simulink model "demo2_supervisory"  (R2024b)
settings: Solver=FixedStepAuto  StartTime=0.0  StopTime=3/60  FixedStep=1/12000  RelTol=1e-3
undefined symbols (not defined in the file): Fault_Inv, GA_th_2, SW, Vd_max, Vd_min, Vdc1, Vdc2, Vdc3, Vdc4, Vdc5, Vq_max, Vq_min
libraries: spsDCVoltageSourceLib x5, spsFullBridgeConverterLib x5, spsSeriesRLCBranchLib x1, spsAlphaBetaZerotodq0Lib x1, spsMeanLib x1, simulink x1, spsVoltageMeasurementLib x1, spspowerguiLib x1
(part 1 of 2)
settings Model: Creator=pgm
settings DataIOCC: ReturnWorkspaceOutputs=off
settings ModelReferenceCC: EnableRefExpFcnMdlSchedulingChecks=on
settings RTWCC: GPUComputeCapability=3.5

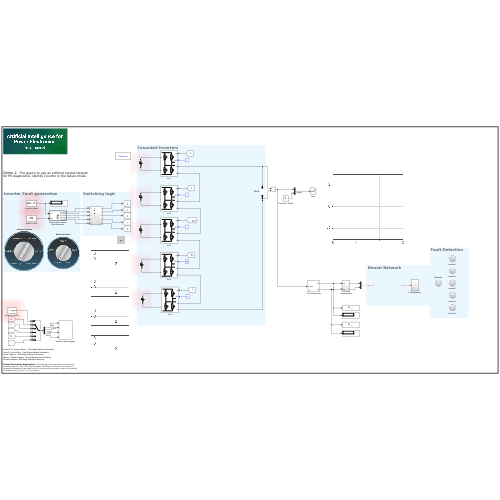
[thumbnail: Simulink's stored preview of the top-level diagram]
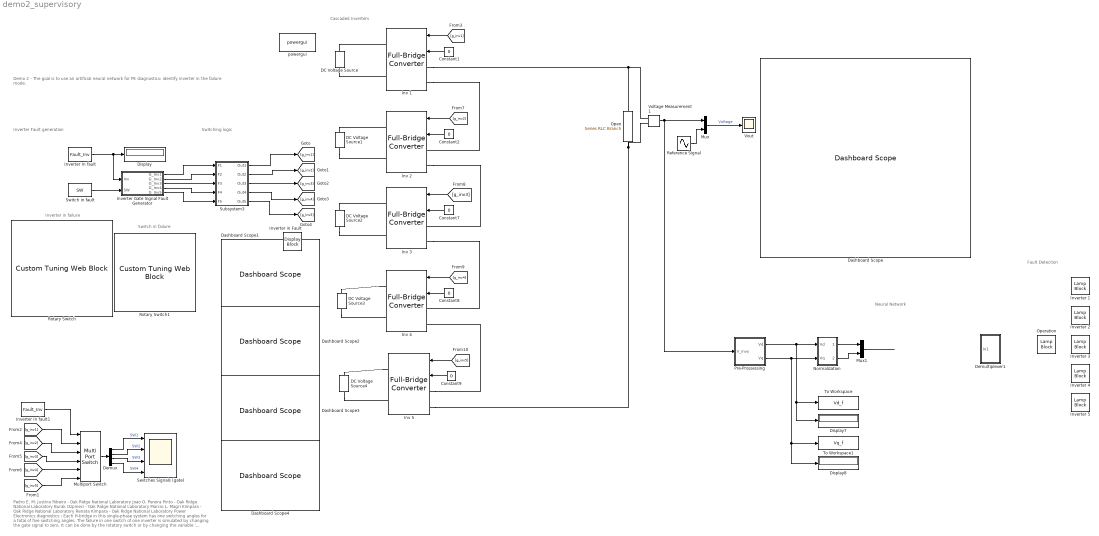
== system demo2_supervisory ==
  note: Inverter in failure
  note: Neural Network
  note: Switching logic
  note: Cascaded Inverters
  note: Inverter Fault generation
  note: Fault Detection
  note: Demo 2 - The goal is to use an artificial neural network for PE diagnostics: identify inverter in the failure mode.
  note: Switch in failure
  note: Pedro E. M. Justino Ribeiro - Oak Ridge National Laboratory
      | Joao O. Pereira Pinto - Oak Ridge National Laboratory
      | Burak Ozpineci - Oak Ridge National Laboratory
      | Marcio L. Magri Kimpara - Oak Ridge National Laboratory
      | Renata Kimpara - Oak Ridge National Laboratory
      |
      | Power Electronics diagnostics : Each H-bridge in this single-phase system has one switching angles for a total of five switching angles. The failure in one switch of one inverter is simulated by changing the gate signal to zero. It can be done by the rotatory switch or by changing the variable ' Fault_Inv' from 1 to 5 in workspace.
  Constant{1..2,7..9} (5 alike) : Constant  Value=0
  DC Voltage Source : spsDCVoltageSourceLib/DC Voltage Source  Amplitude=Vdc1  Measurements=None
  DC Voltage Source1 : spsDCVoltageSourceLib/DC Voltage Source  Amplitude=Vdc2  Measurements=None
  DC Voltage Source2 : spsDCVoltageSourceLib/DC Voltage Source  Amplitude=Vdc3  Measurements=None
  DC Voltage Source3 : spsDCVoltageSourceLib/DC Voltage Source  Amplitude=Vdc4  Measurements=None
  DC Voltage Source4 : spsDCVoltageSourceLib/DC Voltage Source  Amplitude=Vdc5  Measurements=None
  Dashboard Scope : DashboardScope
  Dashboard Scope{1..4} (4 alike) : DashboardScope  TicksPosition=Inside
  Demultiplexer1 : Subsystem
  Demux : Demux
  Display : Display
  Display7 : Display
      settings: Format=short_e
  Display8 : Display
      settings: Format=short_e
  Inv {1..5} (5 alike) : spsFullBridgeConverterLib/Full-Bridge Converter  ModelType=Switching devices  Ron=1e-3  Rs=1e6  Cs=inf  Vforward=[0,0]  Ron_Diode=1e-3  Rs_Diode=1e6  Cs_Diode=inf  Vf_Diode=1e-3  Rs_CurrentSource=inf  Ron_ACsource=1e-3
  Inverter {1..5} (5 alike) : LampBlock  LabelPosition=Hide
  Inverter Gate Signal Fault Generator : MATLAB Function  TreatAsAtomicUnit=on
  Inverter In fault : Constant  Value=Fault_Inv
  Inverter In fault1 : Constant  Value=Fault_Inv
  Inverter in Fault : DisplayBlock  LabelPosition=Hide  Transparency=1
  Multiport Switch : MultiPortSwitch  Inputs=5  DiagnosticForDefault=None  SaturateOnIntegerOverflow=off  InputSameDT=off
  Mux : Mux  Inputs=2
  Mux1 : Mux  Inputs=2
  Normalization : Subsystem
  Open : spsSeriesRLCBranchLib/Series RLC Branch  LConnTagsString=__new0  RConnTagsString=__new0  BranchType=Open circuit  Resistance=50  Inductance=3e-3  SetiL0=off  InitialCurrent=0  Capacitance=400e-6  Setx0=off  InitialVoltage=0  Measurements=None
  "Operation " : LampBlock  LabelPosition=Hide
  Pre-Prossessing : Subsystem  mask{Parameter1=}
      mask prompts: Parameter1 "Transformation"
  Reference Signal : Sin  Amplitude=120*sqrt(2)  Frequency=2*pi*60  SampleTime=0
  Rotary Switch : CustomTuningWebBlock  LabelPosition=Hide  ShowInitialText=on  Configuration="{\"components\":[{\"name\":\"RotarySwitchComponent\",\"settings\":{\"arcAngle\":300,\"arcAngleOffset\":120,\"handle\":{\"size\":[150,150],\"src\":\"data:image\\/svg+xml;base64,PHN2ZyBpZD0iTGF5ZXJfMSIgZGF0YS1uYW1lPSJMYXllciAxIiB4bWxucz0iaHR0cDovL3d3dy53My5vcmcvMjAwMC9zdmciIHhtbG5zOnhsaW5rPSJodHRwOi8vd3d3LnczLm9yZy8xOTk5L3hsaW5rIiB2aWV3Qm94PSIwIDAgMTIxIDEyMSI+PGRlZnM+PHN0eWxlPi5jbHMtMXtmaWxsOnVybCgjbGluZWFyLWdyYWRpZW50KTt9LmNscy0yLC5jbHMtM3tmaWxsOiNkMWQxZDE7fS5jbHMtM3tzdHJva2U6I2I3YjdiNztzdHJva2UtbWl0ZXJsaW1pdDoxMDtzdHJva2Utd2lkdGg6MC4yNXB4O30uY2xzLTR7ZmlsbDojZjMwMDAwO30uY2xzLTV7ZmlsbDojZjIxNzY3O308L3N0eWxlPjxsaW5lYXJHcmFkaWVudCBpZD0ibGluZWFyLWdyYWRpZW50IiB4MT0iNjAuNSIgeTE9IjEyMC41IiB4Mj0iNjAuNSIgeTI9IjAuNSIgZ3JhZGllbnRVbml0cz0idXNlclNwYWNlT25Vc2UiPjxzdG9wIG9mZnNldD0iMCIgc3RvcC1jb2xvcj0iI2QxZDFkMSIvPjxzdG9wIG9mZnNldD0iMC4xIiBzdG9wLWNvbG9yPSIjY2VjZWNlIi8+PHN0b3Agb2Zmc2V0PSIwLjE5IiBzdG9wLWNvbG9yPSIjYzNjM2MzIi8+PHN0b3Agb2Zmc2V0PSIwLjI4IiBzdG9wLWNvbG9yPSIjYjFiMWIxIi8+PHN0b3Agb2Zmc2V0PSIwLjM2IiBzdG9wLWNvbG9yPSIjOTg5ODk4Ii8+PHN0b3Agb2Zmc2V0PSIwLjQ0IiBzdG9wLWNvbG9yPSIjNzg3ODc4Ii8+PHN0b3Agb2Zmc2V0PSIwLjQ2IiBzdG9wLWNvbG9yPSIjNmI2YjZiIi8+PHN0b3Agb2Zmc2V0PSIwLjU0IiBzdG9wLWNvbG9yPSIjNmI2YjZiIi8+PHN0b3Agb2Zmc2V0PSIwLjU2IiBzdG9wLWNvbG9yPSIjNzY3Njc2Ii8+PHN0b3Agb2Zmc2V0PSIwLjY0IiBzdG9wLWNvbG9yPSIjOTc5Nzk3Ii8+PHN0b3Agb2Zmc2V0PSIwLjcyIiBzdG9wLWNvbG9yPSIjYjBiMGIwIi8+PHN0b3Agb2Zmc2V0PSIwLjgxIiBzdG9wLWNvbG9yPSIjYzNjM2MzIi8+PHN0b3Agb2Zmc2V0PSIwLjkiIHN0b3AtY29sb3I9IiNjZGNkY2QiLz48c3RvcCBvZmZzZXQ9IjEiIHN0b3AtY29sb3I9IiNkMWQxZDEiLz48L2xpbmVhckdyYWRpZW50PjwvZGVmcz48Y2lyY2xlIGNsYXNzPSJjbHMtMSIgY3g9IjYwLjUiIGN5PSI2MC41IiByPSI2MCIvPjxwYXRoIGNsYXNzPSJjbHMtMiIgZD0iTTYwLjUsMUE1OS41LDU5LjUsMCwxLDEsMSw2MC41LDU5LjU3LDU5LjU3LDAsMCwxLDYwLjUsMW0wLTFBNjAuNSw2MC41LDAsMSwwLDEyMSw2MC41LDYwLjUsNjAuNSwwLDAsMCw2MC41LDBaIi8+PHJlY3QgY2xhc3M9ImNscy0zIiB4PSIwLjUiIHk9IjUxLjUiIHdpZHRoPSIxMjAiIGhlaWdodD0iMTgiIHJ4PSIzLjA0Ii8+PHJlY3QgY2xhc3M9ImNscy00IiB4PSI1Ljc1IiB5PSI1OC43NSIgd2lkdGg9IjE2IiBoZWlnaHQ9IjMiLz48cGF0aCBjbGFzcz0iY2xzLTUiIGQ9Ik0yMS4yNSw1OS4yNXYyaC0xNXYtMmgxNW0xLTFoLTE3djRoMTd2LTRaIi8+PC9zdmc+\"},\"handleOffset\":[0.00839802927552135,0],\"handleOrientation\":180,\"handlePosition\":[0,0,1,1],\"handleSize\":{\"height\":0.5,\"width\":0.5},\"labelRadius\":0.36,\"position\":[0,0,1,1],\"states\":[{\"Label\":{\"color\":[0,0,0,1],\"icon\":{\"size\":[0,0],\"src\":[],\"srcOrientation\":\"Right\"},\"iconPlacement\":\"left\",\"opacity\":1,\"position\":[0.7345552884615385,0.6796274038461538],\"show\":true,\"text\":{\"content\":\"Normal Op.\",\"font\":\"Helvetica\",\"fontSize\":24}},\"Value\":0},{\"Label\":{\"color\":[0,0,0,1],\"icon\":{\"size\":[0,0],\"src\":[],\"srcOrientation\":\"Right\"},\"iconPlacement\":\"left\",\"opacity\":1,\"position\":[0.35757211538461536,0.7603966346153846],\"show\":true,\"text\":{\"content\":\"Fault Inv1\",\"font\":\"Helvetica\",\"fontSize\":24}},\"Value\":1},{\"Label\":{\"color\":[0,0,0,1],\"icon\":{\"size\":[0,0],\"src\":[],\"srcOrientation\":\"Right\"},\"iconPlacement\":\"left\",\"opacity\":1,\"position\":[0.09603365384615385,0.46033653846153844],\"show\":true,\"text\":{\"content\":\"Fault Inv2\",\"font\":\"Helvetica\",\"fontSize\":24}},\"Value\":2},{\"Label\":{\"color\":[0,0,0,1],\"icon\":{\"size\":[0,0],\"src\":[],\"srcOrientation\":\"Right\"},\"iconPlacement\":\"left\",\"opacity\":1,\"position\":[0.36532451923076925,0.1180889423076923],\"show\":true,\"text\":{\"content\":\"Fault Inv3\",\"font\":\"Helvetica\",\"fontSize\":24}},\"Value\":3},{\"Label\":{\"color\":[0,0,0,1],\"icon\":{\"size\":[0,0],\"src\":[],\"srcOrientation\":\"Right\"},\"iconPlacement\":\"left\",\"opacity\":1,\"position\":[0.7191706730769231,0.19501201923076922],\"show\":true,\"text\":{\"content\":\"Fault Inv4\",\"font\":\"Helvetica\",\"fontSize\":24}},\"Value\":4},{\"Label\":{\"color\":[0,0,0],\"icon\":{\"size\":[1,1],\"src\":\"default\",\"srcOrientation\":\"Right\"},\"iconPlacement\":\"left\",\"opacity\":1,\"position\":[0,0],\"show\":true,\"text\":{\"content\":\"Fault Inv5\",\"fontSize\":14}},\"Value\":5}],\"tickRadius\":0.32}},{\"name\":\"BackgroundImageComponent\",\"settings\":{\"image\":{\"size\":[155,150],\"src\":\"data:image\\/svg+xml;base64,PD94bWwgdmVyc2lvbj0iMS4wIiBlbmNvZGluZz0idXRmLTgiPz4NCjwhLS0gR2VuZXJhdG9yOiBBZG9iZSBJbGx1c3RyYXRvciAyNS4wLjAsIFNWRyBFeHBvcnQgUGx1Zy1JbiAuIFNWRyBWZXJzaW9uOiA2LjAwIEJ1aWxkIDApICAtLT4NCjxzdmcgdmVyc2lvbj0iMS4xIg0KCSBpZD0iTGF5ZXJfMl8xXyIgeG1sbnM6Y2M9Imh0dHA6Ly9jcmVhdGl2ZWNvbW1vbnMub3JnL25zIyIgeG1sbnM6ZGM9Imh0dHA6Ly9wdXJsLm9yZy9kYy9lbGVtZW50cy8xLjEvIiB4bWxuczppbmtzY2FwZT0iaHR0cDovL3d3dy5pbmtzY2FwZS5vcmcv ...(+4184 chars)\",\"srcOrientation\":\"Right\"},\"position\":[0,0,1,1],\"scaleMode\":\"0\"}},{\"name\":\"ForegroundImageComponent\",\"settings\":{\"image\":{\"size\":[0,0],\"src\":\"default\",\"srcOrientation\":[]},\"isForeground\":1,\"position\":[0,0,1,1],\"scaleMode\":\"0\"}}],\"settings\":{\"BindingType\":\"param\",\"backgroundColor\":[0,0,255,\"1\"],\"backgroundOffset\":1,\"enumDataType\":\"\",\"fixedAspectRatio\":\"on\",\"image\":{\"size\":[150,150],\"src\":\"data:image\\/svg+xml;base64,PD94bWwgdmVyc2lvbj0iMS4wIiBlbmNvZGluZz0iVVRGLTgiIHN0YW5kYWxvbmU9Im5vIj8+CjwhLS0gR2VuZXJhdG9yOiBBZG9iZSBJbGx1c3RyYXRvciAxOS4yLjEsIFNWRyBFeHBvcnQgUGx1Zy1JbiAuIFNWRyBWZXJzaW9uOiA2LjAwIEJ1aWxkIDApICAtLT4KCjxzdmcKICAgeG1sbnM6ZGM9Imh0dHA6Ly9wdXJsLm9yZy9kYy9lbGVtZW50cy8xLjEvIgogICB4bWxuczpjYz0iaHR0cDovL2NyZWF0aXZlY29tbW9ucy5vcmcvbnMjIgogICB4bWxuczpyZGY9Imh0dHA6Ly93d3cudzMub3JnLzE5OTkvMDIvMjItcmRmLXN5bnRh ...(+9660 chars)\"},\"showBackgroundColor\":false,\"useEnumDataType\":false,\"variant\":\"rotarySwitch\",\"version\":\"R2024b\"},\"type\":\"RotarySwitch\"}"
  Rotary Switch1 : CustomTuningWebBlock  LabelPosition=Hide  ShowInitialText=on  Configuration="{\"components\":[{\"name\":\"RotarySwitchComponent\",\"settings\":{\"arcAngle\":300,\"arcAngleOffset\":120,\"handle\":{\"size\":[150,150],\"src\":\"data:image\\/svg+xml;base64,PHN2ZyBpZD0iTGF5ZXJfMSIgZGF0YS1uYW1lPSJMYXllciAxIiB4bWxucz0iaHR0cDovL3d3dy53My5vcmcvMjAwMC9zdmciIHhtbG5zOnhsaW5rPSJodHRwOi8vd3d3LnczLm9yZy8xOTk5L3hsaW5rIiB2aWV3Qm94PSIwIDAgMTIxIDEyMSI+PGRlZnM+PHN0eWxlPi5jbHMtMXtmaWxsOnVybCgjbGluZWFyLWdyYWRpZW50KTt9LmNscy0yLC5jbHMtM3tmaWxsOiNkMWQxZDE7fS5jbHMtM3tzdHJva2U6I2I3YjdiNztzdHJva2UtbWl0ZXJsaW1pdDoxMDtzdHJva2Utd2lkdGg6MC4yNXB4O30uY2xzLTR7ZmlsbDojZjMwMDAwO30uY2xzLTV7ZmlsbDojZjIxNzY3O308L3N0eWxlPjxsaW5lYXJHcmFkaWVudCBpZD0ibGluZWFyLWdyYWRpZW50IiB4MT0iNjAuNSIgeTE9IjEyMC41IiB4Mj0iNjAuNSIgeTI9IjAuNSIgZ3JhZGllbnRVbml0cz0idXNlclNwYWNlT25Vc2UiPjxzdG9wIG9mZnNldD0iMCIgc3RvcC1jb2xvcj0iI2QxZDFkMSIvPjxzdG9wIG9mZnNldD0iMC4xIiBzdG9wLWNvbG9yPSIjY2VjZWNlIi8+PHN0b3Agb2Zmc2V0PSIwLjE5IiBzdG9wLWNvbG9yPSIjYzNjM2MzIi8+PHN0b3Agb2Zmc2V0PSIwLjI4IiBzdG9wLWNvbG9yPSIjYjFiMWIxIi8+PHN0b3Agb2Zmc2V0PSIwLjM2IiBzdG9wLWNvbG9yPSIjOTg5ODk4Ii8+PHN0b3Agb2Zmc2V0PSIwLjQ0IiBzdG9wLWNvbG9yPSIjNzg3ODc4Ii8+PHN0b3Agb2Zmc2V0PSIwLjQ2IiBzdG9wLWNvbG9yPSIjNmI2YjZiIi8+PHN0b3Agb2Zmc2V0PSIwLjU0IiBzdG9wLWNvbG9yPSIjNmI2YjZiIi8+PHN0b3Agb2Zmc2V0PSIwLjU2IiBzdG9wLWNvbG9yPSIjNzY3Njc2Ii8+PHN0b3Agb2Zmc2V0PSIwLjY0IiBzdG9wLWNvbG9yPSIjOTc5Nzk3Ii8+PHN0b3Agb2Zmc2V0PSIwLjcyIiBzdG9wLWNvbG9yPSIjYjBiMGIwIi8+PHN0b3Agb2Zmc2V0PSIwLjgxIiBzdG9wLWNvbG9yPSIjYzNjM2MzIi8+PHN0b3Agb2Zmc2V0PSIwLjkiIHN0b3AtY29sb3I9IiNjZGNkY2QiLz48c3RvcCBvZmZzZXQ9IjEiIHN0b3AtY29sb3I9IiNkMWQxZDEiLz48L2xpbmVhckdyYWRpZW50PjwvZGVmcz48Y2lyY2xlIGNsYXNzPSJjbHMtMSIgY3g9IjYwLjUiIGN5PSI2MC41IiByPSI2MCIvPjxwYXRoIGNsYXNzPSJjbHMtMiIgZD0iTTYwLjUsMUE1OS41LDU5LjUsMCwxLDEsMSw2MC41LDU5LjU3LDU5LjU3LDAsMCwxLDYwLjUsMW0wLTFBNjAuNSw2MC41LDAsMSwwLDEyMSw2MC41LDYwLjUsNjAuNSwwLDAsMCw2MC41LDBaIi8+PHJlY3QgY2xhc3M9ImNscy0zIiB4PSIwLjUiIHk9IjUxLjUiIHdpZHRoPSIxMjAiIGhlaWdodD0iMTgiIHJ4PSIzLjA0Ii8+PHJlY3QgY2xhc3M9ImNscy00IiB4PSI1Ljc1IiB5PSI1OC43NSIgd2lkdGg9IjE2IiBoZWlnaHQ9IjMiLz48cGF0aCBjbGFzcz0iY2xzLTUiIGQ9Ik0yMS4yNSw1OS4yNXYyaC0xNXYtMmgxNW0xLTFoLTE3djRoMTd2LTRaIi8+PC9zdmc+\"},\"handleOffset\":[0,0],\"handleOrientation\":180,\"handlePosition\":[0,0,1,1],\"handleSize\":{\"height\":0.5,\"width\":0.5},\"labelRadius\":0.36,\"position\":[0,0,1,1],\"states\":[{\"Label\":{\"color\":[0,0,0,1],\"icon\":{\"size\":[0,0],\"src\":[],\"srcOrientation\":\"Right\"},\"iconPlacement\":\"left\",\"opacity\":1,\"position\":[0.7345552884615385,0.6796274038461538],\"show\":true,\"text\":{\"content\":\"No SW\",\"font\":\"Helvetica\",\"fontSize\":24}},\"Value\":0},{\"Label\":{\"color\":[0,0,0,1],\"icon\":{\"size\":[0,0],\"src\":[],\"srcOrientation\":\"Right\"},\"iconPlacement\":\"left\",\"opacity\":1,\"position\":[0.35757211538461536,0.7603966346153846],\"show\":true,\"text\":{\"content\":\"SW 1\",\"font\":\"Helvetica\",\"fontSize\":24}},\"Value\":1},{\"Label\":{\"color\":[0,0,0,1],\"icon\":{\"size\":[0,0],\"src\":[],\"srcOrientation\":\"Right\"},\"iconPlacement\":\"left\",\"opacity\":1,\"position\":[0.09603365384615385,0.46033653846153844],\"show\":true,\"text\":{\"content\":\"SW 2\",\"font\":\"Helvetica\",\"fontSize\":24}},\"Value\":2},{\"Label\":{\"color\":[0,0,0,1],\"icon\":{\"size\":[0,0],\"src\":[],\"srcOrientation\":\"Right\"},\"iconPlacement\":\"left\",\"opacity\":1,\"position\":[0.36532451923076925,0.1180889423076923],\"show\":true,\"text\":{\"content\":\"SW 3\",\"font\":\"Helvetica\",\"fontSize\":24}},\"Value\":3},{\"Label\":{\"color\":[0,0,0,1],\"icon\":{\"size\":[0,0],\"src\":[],\"srcOrientation\":\"Right\"},\"iconPlacement\":\"left\",\"opacity\":1,\"position\":[0.7191706730769231,0.19501201923076922],\"show\":true,\"text\":{\"content\":\"SW 4\",\"font\":\"Helvetica\",\"fontSize\":24}},\"Value\":4}],\"tickRadius\":0.32}},{\"name\":\"BackgroundImageComponent\",\"settings\":{\"image\":{\"size\":[155,150],\"src\":\"data:image\\/svg+xml;base64,PD94bWwgdmVyc2lvbj0iMS4wIiBlbmNvZGluZz0idXRmLTgiPz4NCjwhLS0gR2VuZXJhdG9yOiBBZG9iZSBJbGx1c3RyYXRvciAyNS4wLjAsIFNWRyBFeHBvcnQgUGx1Zy1JbiAuIFNWRyBWZXJzaW9uOiA2LjAwIEJ1aWxkIDApICAtLT4NCjxzdmcgdmVyc2lvbj0iMS4xIg0KCSBpZD0iTGF5ZXJfMl8xXyIgeG1sbnM6Y2M9Imh0dHA6Ly9jcmVhdGl2ZWNvbW1vbnMub3JnL25zIyIgeG1sbnM6ZGM9Imh0dHA6Ly9wdXJsLm9yZy9kYy9lbGVtZW50cy8xLjEvIiB4bWxuczppbmtzY2FwZT0iaHR0cDovL3d3dy5pbmtzY2FwZS5vcmcv ...(+4184 chars)\",\"srcOrientation\":\"Right\"},\"position\":[0,0,1,1],\"scaleMode\":\"0\"}},{\"name\":\"ForegroundImageComponent\",\"settings\":{\"image\":{\"size\":[0,0],\"src\":\"default\",\"srcOrientation\":[]},\"isForeground\":1,\"position\":[0,0,1,1],\"scaleMode\":\"0\"}}],\"settings\":{\"BindingType\":\"param\",\"backgroundColor\":[0,0,255,\"1\"],\"backgroundOffset\":1,\"enumDataType\":\"\",\"fixedAspectRatio\":\"on\",\"image\":{\"size\":[150,150],\"src\":\"data:image\\/svg+xml;base64,PD94bWwgdmVyc2lvbj0iMS4wIiBlbmNvZGluZz0iVVRGLTgiIHN0YW5kYWxvbmU9Im5vIj8+CjwhLS0gR2VuZXJhdG9yOiBBZG9iZSBJbGx1c3RyYXRvciAxOS4yLjEsIFNWRyBFeHBvcnQgUGx1Zy1JbiAuIFNWRyBWZXJzaW9uOiA2LjAwIEJ1aWxkIDApICAtLT4KCjxzdmcKICAgeG1sbnM6ZGM9Imh0dHA6Ly9wdXJsLm9yZy9kYy9lbGVtZW50cy8xLjEvIgogICB4bWxuczpjYz0iaHR0cDovL2NyZWF0aXZlY29tbW9ucy5vcmcvbnMjIgogICB4bWxuczpyZGY9Imh0dHA6Ly93d3cudzMub3JnLzE5OTkvMDIvMjItcmRmLXN5bnRh ...(+9660 chars)\"},\"showBackgroundColor\":false,\"useEnumDataType\":false,\"variant\":\"rotarySwitch\",\"version\":\"R2024b\"},\"type\":\"RotarySwitch\"}"
  Subsystem3 : Subsystem
  Switch in fault : Constant  Value=SW
  Switches Signals (gate) : Scope  NumInputPorts=4
  To Workspace : ToWorkspace  VariableName=Vd_f  SampleTime=-1
      settings: MaxDataPoints=1
  To Workspace1 : ToWorkspace  VariableName=Vq_f  SampleTime=-1
      settings: MaxDataPoints=1
  Voltage Measurement1 : spsVoltageMeasurementLib/Voltage Measurement  Tag=PoWeRsYsTeMmEaSuReMeNt  PhasorSimulation=off  OutputType=Magnitude  PSBequivalent=0
  Vout : Scope
  powergui : spspowerguiLib/powergui  Priority=1  SimulationMode=Continuous  SampleTime=1e-6  frequency=60  Iterations=50  frequencyindice=0  Pbase=100e6  ErrMax=1e-4  UnitsV=kV  UnitsW=MW  buscounter=0  FunctionMessages=off  echomessages=off  EnableUseOfTLC=off  CurrentSourceSwitches=off  DisableSnubberDevices=off  DisableRonSwitches=off  DisableVfSwitches=off  DisplayEquations=off  AutomaticDiscreteSolvers=off  SolverType=Tustin/Backward Euler (TBE)  Interpol=off  ExternalGateDelay=off  methode=off  Ts=100  x0status=blocks  SPID=on  SwTol=0  HookPort=off  NonlinearTolerance=1e-4  nMaxIteration=100  ContinueOnMaxIteration=off  RestoreLinks=warning  ResistiveCurrentMeasurement=off  Frange=[0:2:500]  Ylog=off  Xlog=on  ShowGrid=off  save=off  variable=ZData  structure=0  ZoomFFT=off  StartTime=0.0  cycles=1  DisplayStyle=1  fundamental=60  FreqAxis=off  MaxFrequency=1000  frequencyindicesteady=1  RmsSteady=1  display=off
  wires:
  Constant1/1 -> Inv 1/2
  Constant2/1 -> Inv 2/2
  [g_inv1] -> Inv 1/1
  [g_inv2] -> Inv 2/1
  [g_inv4] -> Inv 4/1
  [g_inv3] -> Inv 3/1
  Constant8/1 -> Inv 4/2
  Constant7/1 -> Inv 3/2
  Constant9/1 -> Inv 5/2
  [g_inv5] -> Inv 5/1
  Reference Signal/1 -> Mux/2
  Mux/1 -> Vout/1  "Voltage"
  Voltage Measurement1/1 -> Mux/1, Pre-Prossessing/1(V_invs)
  Mux1/1 -> ?
  Pre-Prossessing/2(Vq) -> Normalization/2(Vq), Display8/1, To Workspace1/1
  Pre-Prossessing/1(Vd) -> Normalization/1(Vd), Display7/1, To Workspace/1
  Inverter In fault/1 -> Inverter Gate Signal Fault Generator/1(Inv), Display/1
  Inverter Gate Signal Fault Generator/1(G_Inv1) -> Subsystem3/1(F1)
  Inverter Gate Signal Fault Generator/2(G_Inv2) -> Subsystem3/2(F2)
  Inverter Gate Signal Fault Generator/3(G_Inv3) -> Subsystem3/3(F3)
  Inverter Gate Signal Fault Generator/4(G_Inv4) -> Subsystem3/4(F4)
  Inverter Gate Signal Fault Generator/5(G_Inv5) -> Subsystem3/5(F5)
  Subsystem3/1(Out1) -> [g_inv1]
  Subsystem3/2(Out2) -> [g_inv2]
  Subsystem3/3(Out3) -> [g_inv3]
  Subsystem3/4(Out4) -> [g_inv4]
  Subsystem3/5(Out5) -> [g_inv5]
  [g_inv1] -> Multiport Switch/2
  [g_inv2] -> Multiport Switch/3
  [g_inv3] -> Multiport Switch/4
  [g_inv4] -> Multiport Switch/5
  [g_inv5] -> Multiport Switch/6
  Multiport Switch/1 -> Demux/1
  Demux/1 -> Switches Signals (gate)/1  "SW1"
  Demux/3 -> Switches Signals (gate)/3  "SW3"
  Demux/4 -> Switches Signals (gate)/4  "SW4"
  Demux/2 -> Switches Signals (gate)/2  "SW2"
  Inverter In fault1/1 -> Multiport Switch/1
  Switch in fault/1 -> Inverter Gate Signal Fault Generator/2(SW)
  ? -> Demultiplexer1/1(In1)
  Normalization/2(Out2) -> Mux1/2
  Normalization/1(Out1) -> Mux1/1
  connections:
  DC Voltage Source/RConn1 -- Inv 1/RConn1
  DC Voltage Source/LConn1 -- Inv 1/RConn2
  Inv 2/RConn1 -- DC Voltage Source1/RConn1
  DC Voltage Source1/LConn1 -- Inv 2/RConn2
  Voltage Measurement1/LConn2 -- Inv 5/LConn2 -- Open/RConn1
  Voltage Measurement1/LConn1 -- Inv 1/LConn1 -- Open/LConn1
  Inv 4/RConn1 -- DC Voltage Source3/RConn1
  DC Voltage Source2/LConn1 -- Inv 3/RConn2
  DC Voltage Source3/LConn1 -- Inv 4/RConn2
  DC Voltage Source2/RConn1 -- Inv 3/RConn1
  DC Voltage Source4/LConn1 -- Inv 5/RConn2
  Inv 5/RConn1 -- DC Voltage Source4/RConn1
  Inv 1/LConn2 -- Inv 2/LConn1
  Inv 2/LConn2 -- Inv 3/LConn1
  Inv 3/LConn2 -- Inv 4/LConn1
  Inv 5/LConn1 -- Inv 4/LConn2

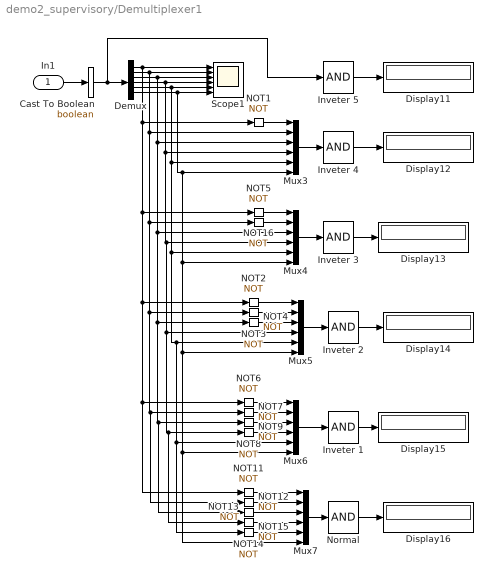
== system demo2_supervisory/Demultiplexer1 ==
  In1 : Inport
  Cast To Boolean : DataTypeConversion  OutDataTypeStr=boolean  SaturateOnIntegerOverflow=off  RndMeth=Floor
  Demux : Demux  Outputs=6
  Display{11..16} (6 alike) : Display
  Inveter {1..5} (5 alike) : Logic  Inputs=1  AllPortsSameDT=off  OutDataTypeStr=boolean
  Mux{3..7} (5 alike) : Mux  Inputs=6
  NOT{1..9,11..16} (15 alike) : Logic  Operator=NOT  IconShape=distinctive  AllPortsSameDT=off  OutDataTypeStr=boolean
  Normal : Logic  Inputs=1  AllPortsSameDT=off  OutDataTypeStr=boolean
  Scope1 : Scope  NumInputPorts=6
  wires:
  In1/1 -> Cast To Boolean/1
  Demux/4 -> Scope1/4, Mux5/4, NOT14/1, NOT9/1, Mux4/4, Mux3/4
  Demux/3 -> Scope1/3, Mux3/3, Mux4/3, NOT13/1, NOT8/1, NOT4/1
  Demux/6 -> Scope1/6, Mux3/6, Mux4/6, Mux5/6, Mux7/6, Mux6/6
  Demux/2 -> Scope1/2, Mux3/2, NOT16/1, NOT3/1, NOT12/1, NOT7/1
  NOT9/1 -> Mux6/4
  Demux/1 -> Scope1/1, NOT1/1, NOT5/1, NOT2/1, NOT11/1, NOT6/1
  Mux3/1 -> Inveter 4/1
  Inveter 4/1 -> Display12/1
  Mux6/1 -> Inveter 1/1
  Inveter 1/1 -> Display15/1
  Mux7/1 -> Normal/1
  Normal/1 -> Display16/1
  Mux4/1 -> Inveter 3/1
  Inveter 3/1 -> Display13/1
  Inveter 2/1 -> Display14/1
  Inveter 5/1 -> Display11/1
  Cast To Boolean/1 -> Inveter 5/1, Demux/1
  Mux5/1 -> Inveter 2/1
  NOT1/1 -> Mux3/1
  NOT5/1 -> Mux4/1
  NOT16/1 -> Mux4/2
  NOT2/1 -> Mux5/1
  NOT3/1 -> Mux5/2
  NOT4/1 -> Mux5/3
  NOT6/1 -> Mux6/1
  NOT7/1 -> Mux6/2
  NOT8/1 -> Mux6/3
  Demux/5 -> Scope1/5, Mux3/5, Mux4/5, Mux5/5, Mux6/5, NOT15/1
  NOT11/1 -> Mux7/1
  NOT12/1 -> Mux7/2
  NOT13/1 -> Mux7/3
  NOT14/1 -> Mux7/4
  NOT15/1 -> Mux7/5

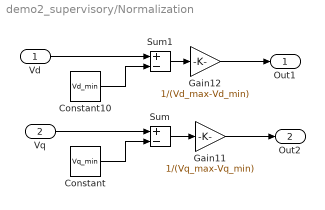
== system demo2_supervisory/Normalization ==
  Vd : Inport
  Vq : Inport  Port=2
  Constant : Constant  Value=Vq_min
  Constant10 : Constant  Value=Vd_min
  Gain11 : Gain  Gain=1/(Vq_max-Vq_min)
  Gain12 : Gain  Gain=1/(Vd_max-Vd_min)
  Sum : Sum  Inputs=+-
  Sum1 : Sum  Inputs=+-
  Out1 : Outport
  Out2 : Outport  Port=2
  wires:
  Gain12/1 -> Out1/1
  Constant/1 -> Sum/2
  Sum1/1 -> Gain12/1
  Vd/1 -> Sum1/1
  Constant10/1 -> Sum1/2
  Sum/1 -> Gain11/1
  Gain11/1 -> Out2/1
  Vq/1 -> Sum/1

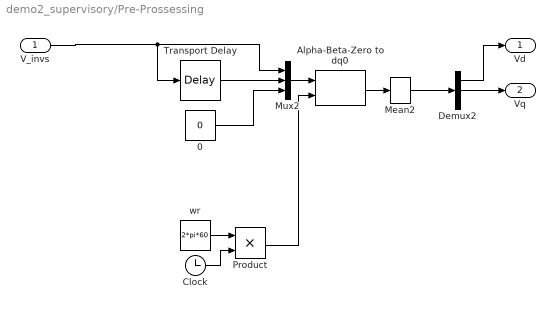
== system demo2_supervisory/Pre-Prossessing ==
  V_invs : Inport
  0 : Constant  Value=0
  Alpha-Beta-Zero to dq0 : spsAlphaBetaZerotodq0Lib/Alpha-Beta-Zero to dq0  Alignment=Aligned with phase A axis
  Clock : Clock
  Demux2 : Demux  Outputs=3
  Mean2 : spsMeanLib/Mean  Freq=60  Vinit=0  Ts=0
  Mux2 : Mux  Inputs=3
  Product : Product
  Transport Delay : TransportDelay  DelayTime=(1/60)/4
  wr : Constant  Value=2*pi*60
  Vd : Outport
  Vq : Outport  Port=2
  wires:
  Mux2/1 -> Alpha-Beta-Zero to dq0/1
  Mean2/1 -> Demux2/1
  Demux2/2 -> Vq/1
  Product/1 -> Alpha-Beta-Zero to dq0/2
  Transport Delay/1 -> Mux2/2
  wr/1 -> Product/1
  Clock/1 -> Product/2
  0/1 -> Mux2/3
  Alpha-Beta-Zero to dq0/1 -> Mean2/1
  V_invs/1 -> Mux2/1, Transport Delay/1
  Demux2/1 -> Vd/1
